simulink model "MBD_Merge"  (R2021b)
settings: Solver=FixedStepDiscrete  StartTime=0.0  StopTime=10.0  FixedStep=0.01  RelTol=1e-3
libraries: simulink x1
settings Model: Creator=waleed.elshemy  LastModifiedBy=waleed.elshemy

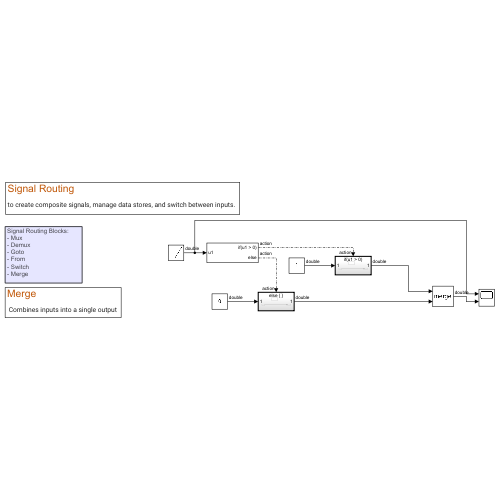
[thumbnail: Simulink's stored preview of the top-level diagram]
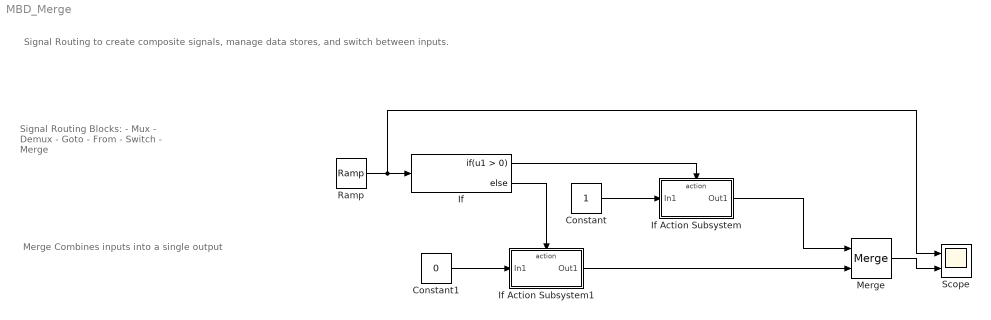
== system MBD_Merge ==
  note: Signal Routing
      | to create composite signals, manage data stores, and switch between inputs.
  note: Signal Routing Blocks:
      | - Mux
      | - Demux
      | - Goto
      | - From
      | - Switch
      | - Merge
  note: Merge
      | Combines inputs into a single output
  Constant : Constant
  Constant1 : Constant  Value=0
  If : If
  If Action Subsystem : Subsystem  TreatAsAtomicUnit=on
  If Action Subsystem1 : Subsystem  TreatAsAtomicUnit=on
  Merge : Merge
  Ramp : simulink/Sources/Ramp  slope=1  start=0  InitialOutput=-5
  Scope : Scope  NumInputPorts=2
  wires:
  If/1 -> If Action Subsystem/Action
  If/2 -> If Action Subsystem1/Action
  Constant/1 -> If Action Subsystem/1(In1)
  Constant1/1 -> If Action Subsystem1/1(In1)
  Ramp/1 -> Scope/1, If/1
  If Action Subsystem/1(Out1) -> Merge/1
  If Action Subsystem1/1(Out1) -> Merge/2
  Merge/1 -> Scope/2

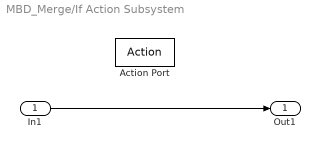
== system MBD_Merge/If Action Subsystem ==
  In1 : Inport
  Action Port : ActionPort  ActionPortLabel=if(u1 > 0)
  Out1 : Outport
  wires:
  In1/1 -> Out1/1

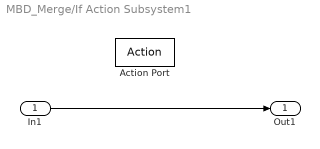
== system MBD_Merge/If Action Subsystem1 ==
  In1 : Inport
  Action Port : ActionPort  ActionPortLabel=else
  Out1 : Outport
  wires:
  In1/1 -> Out1/1
